simulink model "DM_overflow"  (R2021b)
settings: Solver=FixedStepAuto  StartTime=0.0  StopTime=sim_duration  FixedStep=0.1  RelTol=1e-3
model workspace: external: MAT-File C:\Users\jimmy\Desktop\61508010.mat (data not in the file)
undefined symbols (not defined in the file or in its folder): Base_power, efficiency_3D1, efficiency_3D3, efficiency_speed_3D1, efficiency_speed_3D3, efficiency_torque_3D1, efficiency_torque_3D3, f_d, f_tire_friction, f_tire_speed, g, gear_efficiency, Init_capacity, Max_T_3D1, OCV, OCV_SOC, r_mass, Regen_fraction, Regen_speed, SOC_init, SOC_min, Stop_speed, Torque_curve_speed_3D1, Torque_curve_speed_3D3, Torque_curve_torque_3D1, Torque_curve_torque_3D3, Vehicle_weight, Wheel_radius
libraries: fl_lib x18, nesl_utility x10, sdl_lib x7, simulink x2
settings Model: Creator=jimmy  LastModifiedBy=jimmy
settings DebuggingCC: UnderSpecifiedDimensionMsg=warning
settings SimscapeCC: ExplicitSolverDiagnosticOptions=none

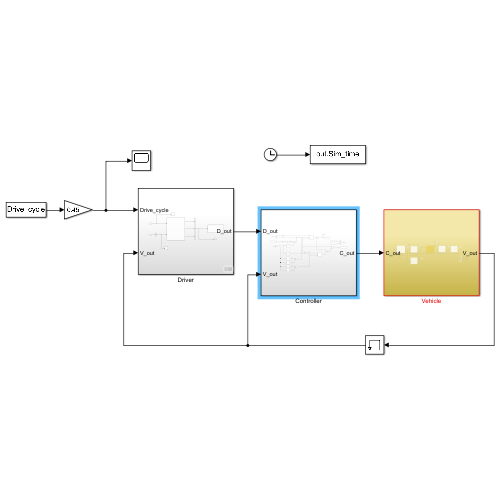
[thumbnail: Simulink's stored preview of the top-level diagram]
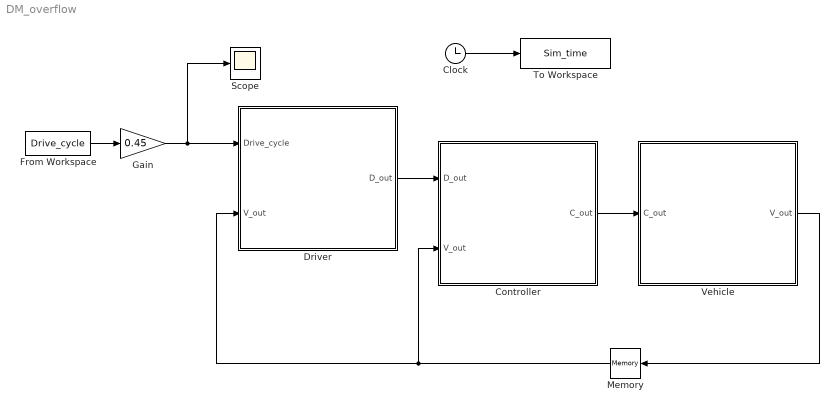
== system DM_overflow ==
  Clock : Clock
  Controller : Subsystem
  Driver : Subsystem
  From Workspace : FromWorkspace  VariableName=Drive_cycle
  Gain : Gain  Gain=0.45
  Memory : Memory  InheritSampleTime=on  LinearizeMemory=on  LinearizeAsDelay=on
  Scope : Scope
  To Workspace : ToWorkspace  VariableName=Sim_time  SaveFormat=Timeseries  SampleTime=-1
  Vehicle : Subsystem
  wires:
  Vehicle/1(V_out) -> Memory/1
  Controller/1(C_out) -> Vehicle/1(C_out)
  Memory/1 -> Controller/2(V_out), Driver/2(V_out)
  Clock/1 -> To Workspace/1
  Driver/1(D_out) -> Controller/1(D_out)
  From Workspace/1 -> Gain/1
  Gain/1 -> Scope/1, Driver/1(Drive_cycle)

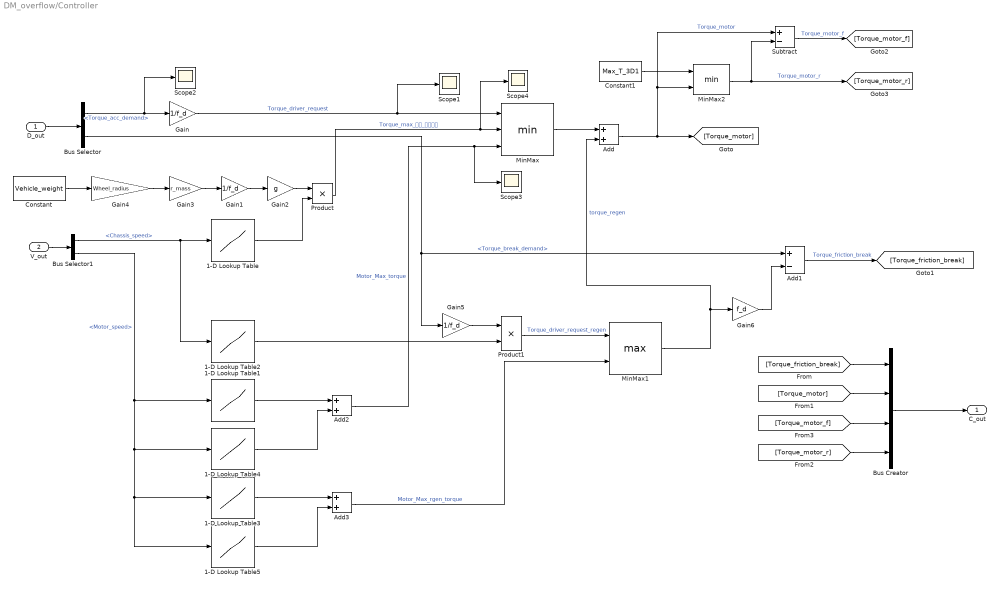
== system DM_overflow/Controller ==
  D_out : Inport
  V_out : Inport  Port=2
  1-D Lookup Table : Lookup_n-D  NumberOfTableDimensions=1  BreakpointsForDimension1=f_tire_speed  Table=f_tire_friction  InternalRulePriority=Speed  RndMeth=Simplest  InputSameDT=on
  1-D Lookup Table1 : Lookup_n-D  NumberOfTableDimensions=1  BreakpointsForDimension1=Torque_curve_speed_3D1  Table=Torque_curve_torque_3D1  InternalRulePriority=Speed  RndMeth=Simplest  InputSameDT=on
  1-D Lookup Table2 : Lookup_n-D  NumberOfTableDimensions=1  BreakpointsForDimension1=Regen_speed  Table=Regen_fraction  InternalRulePriority=Speed  RndMeth=Simplest  InputSameDT=on
  1-D Lookup Table3 : Lookup_n-D  NumberOfTableDimensions=1  BreakpointsForDimension1=Torque_curve_speed_3D1  Table=-Torque_curve_torque_3D1  InternalRulePriority=Speed  RndMeth=Simplest  InputSameDT=on
  1-D Lookup Table4 : Lookup_n-D  NumberOfTableDimensions=1  BreakpointsForDimension1=Torque_curve_speed_3D3  Table=Torque_curve_torque_3D3  InternalRulePriority=Speed  RndMeth=Simplest  InputSameDT=on
  1-D Lookup Table5 : Lookup_n-D  NumberOfTableDimensions=1  BreakpointsForDimension1=Torque_curve_speed_3D3  Table=-Torque_curve_torque_3D3  InternalRulePriority=Speed  RndMeth=Simplest  InputSameDT=on
  Add : Sum
  Add1 : Sum  Inputs=+-
  Add2 : Sum
  Add3 : Sum
  Bus Creator : BusCreator  Inputs=4
  Bus Selector : BusSelector  OutputSignals=Torque_acc_demand,Torque_break_demand
  Bus Selector1 : BusSelector  OutputSignals=Chassis_speed,signal3.Motor_speed
  Constant : Constant  Value=Vehicle_weight
  Constant1 : Constant  Value=Max_T_3D1
  Gain : Gain  Gain=1/f_d
  Gain1 : Gain  Gain=1/f_d
  Gain2 : Gain  Gain=g
  Gain3 : Gain  Gain=r_mass
  Gain4 : Gain  Gain=Wheel_radius
  Gain5 : Gain  Gain=1/f_d
  Gain6 : Gain  Gain=f_d
  MinMax : MinMax  Inputs=3
  MinMax1 : MinMax  Function=max  Inputs=2
  MinMax2 : MinMax  Inputs=2
  Product : Product
  Product1 : Product
  Scope{1..4} (4 alike) : Scope
  Subtract : Sum  Inputs=+-
  C_out : Outport
  wires:
  D_out/1 -> Bus Selector/1
  Bus Selector/1 -> Scope2/1, Gain/1  "<Torque_acc_demand>"
  Bus Selector/2 -> Add1/1, Gain5/1  "<Torque_break_demand>"
  Gain/1 -> Scope1/1, MinMax/1  "Torque_driver_request"
  Constant/1 -> Gain4/1
  Gain4/1 -> Gain3/1
  Gain3/1 -> Gain1/1
  Gain1/1 -> Gain2/1
  1-D Lookup Table/1 -> Product/2
  Bus Selector1/1 -> 1-D Lookup Table2/1, 1-D Lookup Table/1  "<Chassis_speed>"
  Gain2/1 -> Product/1
  V_out/1 -> Bus Selector1/1
  Product/1 -> Scope4/1, MinMax/2  "Torque_max_𝑛𝑜_𝑠𝑙𝑖𝑝"
  MinMax/1 -> Add/1
  Bus Selector1/2 -> 1-D Lookup Table1/1, 1-D Lookup Table4/1, 1-D Lookup Table3/1, 1-D Lookup Table5/1  "<Motor_speed>"
  Gain5/1 -> Product1/1
  1-D Lookup Table2/1 -> Product1/2
  Product1/1 -> MinMax1/1  "Torque_driver_request_regen"
  MinMax1/1 -> Gain6/1, Add/2  "torque_regen"
  Add/1 -> Subtract/1, MinMax2/2, [Torque_motor]  "Torque_motor"
  Gain6/1 -> Add1/2
  Add1/1 -> [Torque_friction_break]  "Torque_friction_break"
  [Torque_motor] -> Bus Creator/2
  [Torque_friction_break] -> Bus Creator/1
  Bus Creator/1 -> C_out/1
  Add3/1 -> MinMax1/2  "Motor_Max_rgen_torque"
  Add2/1 -> Scope3/1, MinMax/3  "Motor_Max_torque"
  1-D Lookup Table1/1 -> Add2/1
  1-D Lookup Table3/1 -> Add3/1
  1-D Lookup Table4/1 -> Add2/2
  1-D Lookup Table5/1 -> Add3/2
  [Torque_motor_f] -> Bus Creator/3
  [Torque_motor_r] -> Bus Creator/4
  Constant1/1 -> MinMax2/1
  MinMax2/1 -> Subtract/2, [Torque_motor_r]  "Torque_motor_r"
  Subtract/1 -> [Torque_motor_f]  "Torque_motor_f"

== system DM_overflow/Driver ==
  Drive_cycle : Inport
  V_out : Inport  Port=2
  Bus Creator : BusCreator  Inputs=3
  Bus Selector : BusSelector  OutputSignals=Chassis_speed
  Plant : Subsystem
  Scope : Scope
  Scope1 : Scope
  To workspace : Subsystem
  D_out : Outport
  wires:
  Drive_cycle/1 -> Scope/1, Plant/1(Drive_cycle)
  V_out/1 -> Bus Selector/1
  Bus Selector/1 -> Scope1/1, Plant/2(Chasis_speed)  "<Chassis_speed>"
  Plant/1(Linear_speed_demand) -> Bus Creator/1
  Plant/2(Torque_acc_demand) -> Bus Creator/2
  Plant/3(Torque_break_demand) -> Bus Creator/3
  Bus Creator/1 -> D_out/1, To workspace/1(In1)

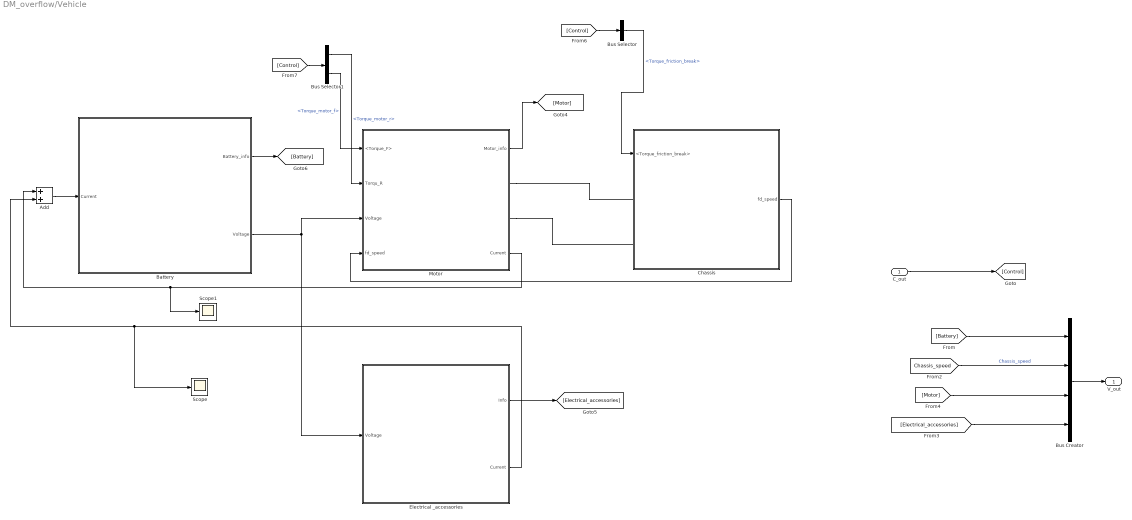
== system DM_overflow/Vehicle ==
  C_out : Inport
  Add : Sum
  Battery : Subsystem
  Bus Creator : BusCreator  Inputs=4
  Bus Selector : BusSelector  OutputSignals=Torque_friction_break
  Bus Selector1 : BusSelector  OutputSignals=Torque_motor_r,Torque_motor_f
  Chassis : Subsystem
  Electrical _accessories : Subsystem
  Motor : Subsystem
      settings: PortSchema="{\"entries\":[{\"content\":{\"sides\":[{\"content\":{\"connectorIds\":[\"In1\",\"In2\",\"In3\",\"In4\"]},\"type\":\"ConnectorPlacement.EquallySpacedRectSide\",\"uuid\":\"41143f5e-7686-4338-be62-9090af3e7fda\"},{\"content\":{\"connectorIds\":[\"Out1\",\"RConn1\",\"RConn2\",\"Out2\"],\"side\":\"RIGHT\"},\"type\":\"ConnectorPlacement.EquallySpacedRectSide\",\"uuid\":\"80376a3c-2384-4fc0-8e0f-19ad3c35f516\"},{\"content\":{\"connectorIds\":[],\"side\":\"TOP\"},\"type\":\"ConnectorPlacement.EquallySpacedRectSide\",\"uuid\":\"cc882acb-b744-4941-b3e2-8b777c6c03a1\"}]},\"type\":\"ConnectorPlacement.EquallySpacedConnector\",\"uuid\":\"b67d3583-afb0-4dd1-8124-18a93feb2c2f\"}],\"packageUris\":[\"http://schema.mathworks.com/mf0/Connector/R2020b\"],\"version\":\"1.0\"}"
  Scope : Scope
  Scope1 : Scope
  V_out : Outport
  wires:
  Bus Creator/1 -> V_out/1
  [Battery] -> Bus Creator/1
  [Chassis_speed] -> Bus Creator/2  "Chassis_speed"
  [Motor] -> Bus Creator/3
  [Electrical_accessories] -> Bus Creator/4
  C_out/1 -> [Control]
  Battery/2(Voltage) -> Motor/3(Voltage), Electrical _accessories/1(Voltage)
  Motor/2(Current) -> Scope1/1, Add/1
  Motor/1(Motor_info) -> [Motor]
  [Control] -> Bus Selector1/1
  Bus Selector1/1 -> Motor/2(Torqu_R)  "<Torque_motor_r>"
  Add/1 -> Battery/1(Current)
  Electrical _accessories/2(Current) -> Scope/1, Add/2
  Electrical _accessories/1(Info) -> [Electrical_accessories]
  Battery/1(Battery_info) -> [Battery]
  Chassis/1(fd_speed) -> Motor/4(fd_speed)
  [Control] -> Bus Selector/1
  Bus Selector/1 -> Chassis/1(<Torque_friction_break>)  "<Torque_friction_break>"
  Bus Selector1/2 -> Motor/1(<Torque_F>)  "<Torque_motor_f>"
  connections:
  Motor/RConn1 -- Chassis/LConn1
  Motor/RConn2 -- Chassis/LConn2

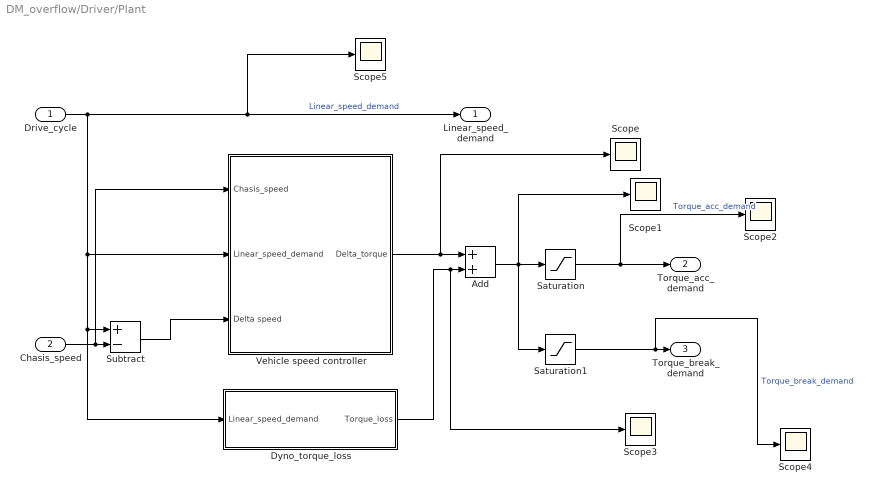
== system DM_overflow/Driver/Plant ==
  Drive_cycle : Inport
  Chasis_speed : Inport  Port=2
  Add : Sum
  Dyno_torque_loss : Subsystem
  Saturation : Saturate  UpperLimit=inf  LowerLimit=0
  Saturation1 : Saturate  UpperLimit=0  LowerLimit=-inf
  Scope{,1..5} (6 alike) : Scope
  Subtract : Sum  Inputs=+-
  Vehicle speed controller : Subsystem
  Linear_speed_demand : Outport
  Torque_acc_demand : Outport  Port=2
  Torque_break_demand : Outport  Port=3
  wires:
  Drive_cycle/1 -> Vehicle speed controller/2(Linear_speed_demand), Dyno_torque_loss/1(Linear_speed_demand), Subtract/1, Scope5/1, Linear_speed_demand/1  "Linear_speed_demand"
  Chasis_speed/1 -> Vehicle speed controller/1(Chasis_speed), Subtract/2
  Subtract/1 -> Vehicle speed controller/3(Delta speed)
  Vehicle speed controller/1(Delta_torque) -> Scope/1, Add/1
  Dyno_torque_loss/1(Torque_loss) -> Scope3/1, Add/2
  Add/1 -> Saturation1/1, Scope1/1, Saturation/1
  Saturation/1 -> Scope2/1, Torque_acc_demand/1  "Torque_acc_demand"
  Saturation1/1 -> Scope4/1, Torque_break_demand/1  "Torque_break_demand"

== system DM_overflow/Driver/To workspace ==
  In1 : Inport
  Bus Selector : BusSelector  OutputSignals=Linear_speed_demand,Torque_acc_demand,Torque_break_demand
  To Workspace : ToWorkspace  VariableName=Linear_speed_demand  SampleTime=0.1
      settings: Decimation=10  Save2DSignal=2-D array (concatenate along first dimension)
  To Workspace2 : ToWorkspace  VariableName=Torque_break_demand  SampleTime=-1
      settings: Decimation=10
  To Workspace3 : ToWorkspace  VariableName=Torque_acc_demand  SampleTime=-1
      settings: Decimation=10
  wires:
  In1/1 -> Bus Selector/1
  Bus Selector/1 -> To Workspace/1  "<Linear_speed_demand>"
  Bus Selector/2 -> To Workspace3/1  "<Torque_acc_demand>"
  Bus Selector/3 -> To Workspace2/1  "<Torque_break_demand>"

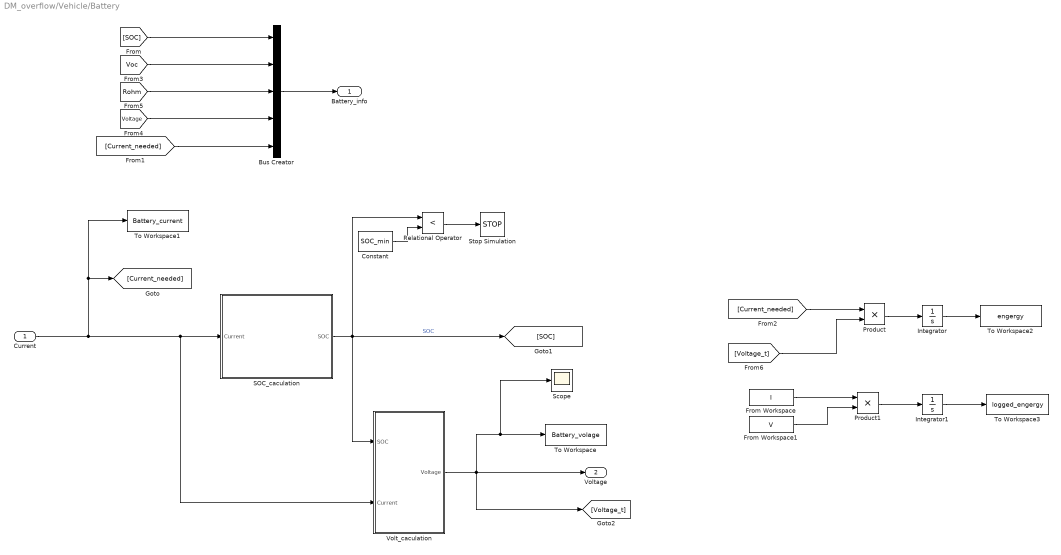
== system DM_overflow/Vehicle/Battery ==
  Current : Inport
  Bus Creator : BusCreator  Inputs=5
  Constant : Constant  Value=SOC_min
  From Workspace : FromWorkspace  VariableName=I
  From Workspace1 : FromWorkspace  VariableName=V
  Integrator : Integrator
  Integrator1 : Integrator
  Product : Product
  Product1 : Product
  Relational Operator : RelationalOperator  Operator=<  OutDataTypeStr=boolean  RndMeth=Simplest
  SOC_caculation : Subsystem
  Scope : Scope
  Stop Simulation : Stop
  To Workspace : ToWorkspace  VariableName=Battery_volage  SampleTime=0.1
  To Workspace1 : ToWorkspace  VariableName=Battery_current  SampleTime=0.1
  To Workspace2 : ToWorkspace  VariableName=engergy  SampleTime=-1
  To Workspace3 : ToWorkspace  VariableName=logged_engergy  SampleTime=-1
  Volt_caculation : Subsystem
  Battery_info : Outport
  Voltage : Outport  Port=2
  wires:
  Current/1 -> To Workspace1/1, [Current_needed], Volt_caculation/2(Current), SOC_caculation/1(Current)
  SOC_caculation/1(SOC) -> Volt_caculation/1(SOC), Relational Operator/1, [SOC]  "SOC"
  Constant/1 -> Relational Operator/2
  Relational Operator/1 -> Stop Simulation/1
  Volt_caculation/1(Voltage) -> [Voltage_t], Scope/1, To Workspace/1, Voltage/1
  Bus Creator/1 -> Battery_info/1
  [Current_needed] -> Bus Creator/5
  [SOC] -> Bus Creator/1
  [Voc] -> Bus Creator/2
  [Rohm] -> Bus Creator/3
  [Voltage] -> Bus Creator/4
  [Voltage_t] -> Product/2
  [Current_needed] -> Product/1
  Product/1 -> Integrator/1
  Integrator/1 -> To Workspace2/1
  From Workspace/1 -> Product1/1
  From Workspace1/1 -> Product1/2
  Product1/1 -> Integrator1/1
  Integrator1/1 -> To Workspace3/1

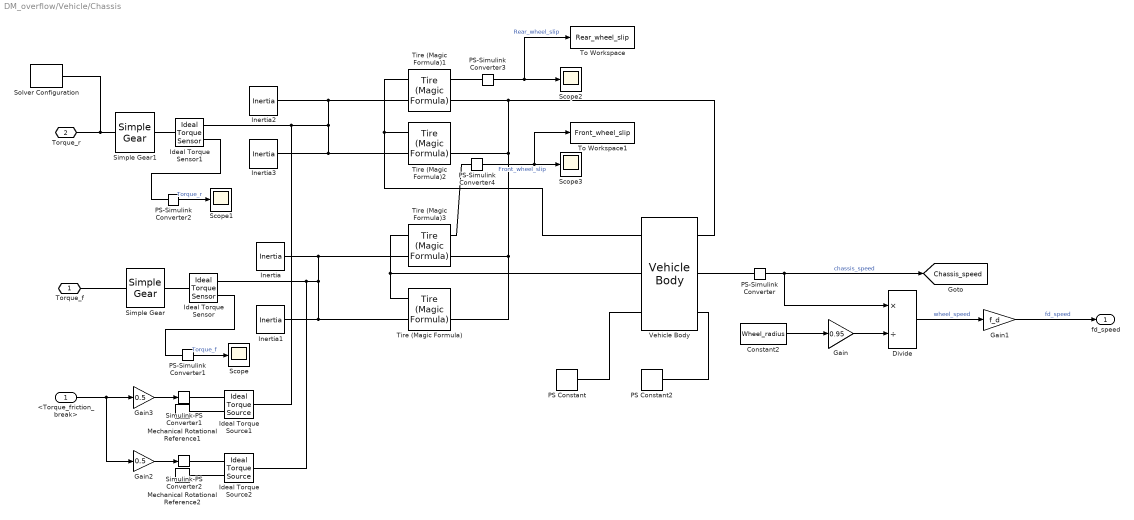
== system DM_overflow/Vehicle/Chassis ==
  <Torque_friction_break> : Inport
  Constant2 : Constant  Value=Wheel_radius
  Divide : Product  Inputs=*/
  Gain : Gain  Gain=0.95
  Gain1 : Gain  Gain=f_d
  Gain2 : Gain  Gain=0.5
  Gain3 : Gain  Gain=0.5
  Ideal Torque Sensor : fl_lib/Mechanical/Mechanical Sensors/Ideal Torque Sensor
  Ideal Torque Sensor1 : fl_lib/Mechanical/Mechanical Sensors/Ideal Torque Sensor
  Ideal Torque Source1 : fl_lib/Mechanical/Mechanical Sources/Ideal Torque Source
  Ideal Torque Source2 : fl_lib/Mechanical/Mechanical Sources/Ideal Torque Source
  Inertia{,1..3} (4 alike) : fl_lib/Mechanical/Rotational Elements/Inertia  inertia=1 kg*m^2  num_ports=foundation.enum.numPorts2.one  w_specify=off  w_priority=High  w=0 rad/s  w_nominal_specify=off  w_nominal_unit=rad/s  w_nominal_value=1  t_specify=off  t_priority=None  t=0 N*m  t_nominal_specify=off  t_nominal_unit=N*m  t_nominal_value=1
  Mechanical Rotational Reference1 : fl_lib/Mechanical/Rotational Elements/Mechanical Rotational Reference
  Mechanical Rotational Reference2 : fl_lib/Mechanical/Rotational Elements/Mechanical Rotational Reference
  PS Constant : fl_lib/Physical Signals/Sources/PS Constant  constant=0
  PS Constant2 : fl_lib/Physical Signals/Sources/PS Constant  constant=5 m/s
  PS-Simulink Converter{,1..4} (5 alike) : nesl_utility/PS-Simulink Converter  PhysicalDomain=network_engine_domain  SubClassName=ps_output  LeftPortType=input  RightPortType=output  PseudoPeriodic=off  Frequencies=[]  Unit=inherit  AffineConversion=off
      settings: SourceProductBaseCode=PW,SS
  Scope{,1..3} (4 alike) : Scope
  Simple Gear : sdl_lib/Gears/Simple Gear  ratio=f_d  rotation_direction=sdl.enum.shaftOutputDirection.same  friction_model=sdl.enum.gear_efficiencies_load.off  T_noload=0.1 N*m  T_nom=5 N*m  efficiency_nom=0.8  efficiency=0.8  temperature_TLU=[280, 300, 320] K  load_TLU=[1, 5, 10] N*m  efficiency_TLU=[.95, .9, .85]  efficiency_TLU2=[.85, .8, .75; .95, .9, .85; .85, .8, .7]  w_thr=0.01 rad/s  pwr_thr=0.001 W  backlash_model=sdl.enum.backlashModel.Off  backlash_distance=1e-3 mm  x0=0 mm  r_base=0.1 m  hardstop_model=simscape.enum.hardstop.smooth  transition=1e-4 mm  backlash_stiffness=1e7 N/m  backlash_damping=1e6 N/(m/s)  e=0  v_tol=0.001 m/s  mu_visc=[0, 0] N*m/(rad/s)  enable_faults=simscape.enum.onoff.off  efficiency_fault=0.05  external_fault=simscape.enum.onoff.off  temporal_fault=simscape.enum.onoff.off  fault_time=5 s  fault_angles=pi / 12 rad  report_fault=simscape.enum.assert.action.none  thermal_mass=50 J/K  temperature_specify=off  temperature_priority=High  temperature=300 K  temperature_nominal_specify=off  temperature_nominal_unit=K  temperature_nominal_value=1  x_backlash_specify=off  x_backlash_priority=None  x_backlash=0 mm  x_backlash_nominal_specify=off  x_backlash_nominal_unit=mm  x_backlash_nominal_value=1  f_hardstop_specify=off  f_hardstop_priority=None  f_hardstop=0 N  f_hardstop_nominal_specify=off  f_hardstop_nominal_unit=N  f_hardstop_nominal_value=1  v_backlash_specify=off  v_backlash_priority=None  v_backlash=0 m/s  v_backlash_nominal_specify=off  v_backlash_nominal_unit=m/s  v_backlash_nominal_value=1
  Simple Gear1 : sdl_lib/Gears/Simple Gear  ratio=f_d  rotation_direction=sdl.enum.shaftOutputDirection.same  friction_model=sdl.enum.gear_efficiencies_load.off  T_noload=0.1 N*m  T_nom=5 N*m  efficiency_nom=0.8  efficiency=0.8  temperature_TLU=[280, 300, 320] K  load_TLU=[1, 5, 10] N*m  efficiency_TLU=[.95, .9, .85]  efficiency_TLU2=[.85, .8, .75; .95, .9, .85; .85, .8, .7]  w_thr=0.01 rad/s  pwr_thr=0.001 W  backlash_model=sdl.enum.backlashModel.Off  backlash_distance=1e-3 mm  x0=0 mm  r_base=0.1 m  hardstop_model=simscape.enum.hardstop.smooth  transition=1e-4 mm  backlash_stiffness=1e7 N/m  backlash_damping=1e6 N/(m/s)  e=0  v_tol=0.001 m/s  mu_visc=[0, 0] N*m/(rad/s)  enable_faults=simscape.enum.onoff.off  efficiency_fault=0.05  external_fault=simscape.enum.onoff.off  temporal_fault=simscape.enum.onoff.off  fault_time=5 s  fault_angles=pi / 12 rad  report_fault=simscape.enum.assert.action.none  thermal_mass=50 J/K  temperature_specify=off  temperature_priority=High  temperature=300 K  temperature_nominal_specify=off  temperature_nominal_unit=K  temperature_nominal_value=1  x_backlash_specify=off  x_backlash_priority=None  x_backlash=0 mm  x_backlash_nominal_specify=off  x_backlash_nominal_unit=mm  x_backlash_nominal_value=1  f_hardstop_specify=off  f_hardstop_priority=None  f_hardstop=0 N  f_hardstop_nominal_specify=off  f_hardstop_nominal_unit=N  f_hardstop_nominal_value=1  v_backlash_specify=off  v_backlash_priority=None  v_backlash=0 m/s  v_backlash_nominal_specify=off  v_backlash_nominal_unit=m/s  v_backlash_nominal_value=1
  Simulink-PS Converter1 : nesl_utility/Simulink-PS Converter  PhysicalDomain=network_engine_domain  SubClassName=ps_input  LeftPortType=input  RightPortType=output  PseudoPeriodic=off  Frequencies=[]  NoiseDistribution=none  NoiseParameters=[]  Unit=N*m  AffineConversion=off  FilteringAndDerivatives=provide  SimscapeFilterOrder=2  InputFilterTimeConstant=0.001  UdotUserProvided=0
      settings: SourceProductBaseCode=PW,SS
  Simulink-PS Converter2 : nesl_utility/Simulink-PS Converter  PhysicalDomain=network_engine_domain  SubClassName=ps_input  LeftPortType=input  RightPortType=output  PseudoPeriodic=off  Frequencies=[]  NoiseDistribution=none  NoiseParameters=[]  Unit=N*m  AffineConversion=off  FilteringAndDerivatives=provide  SimscapeFilterOrder=2  InputFilterTimeConstant=0.001  UdotUserProvided=0
      settings: SourceProductBaseCode=PW,SS
  Solver Configuration : nesl_utility/Solver Configuration  PhysicalDomain=network_engine_domain  SubClassName=solver  LeftPortType=input  RightPortType=generic  Tones=[]  Harmonics=[]  SimulateNoise=off  Profile=off  UseLocalSampling=off  EnableSwitchedLinearOptims=on  FrequencyDomain=off  UseCCode=off  RelTol=0.001  AbsTol=1e-06  MinStep=1e-09  ToWorkspace=off  RevertToSquareIcSolve=off  NumHomotopyIterations=100  PhasorMode=off  PhasorModeNumHarmonics=1  DoDC=off  ResidualTolerance=1e-06  UseLocalSolver=off  LocalSolverChoice=NE_BACKWARD_EULER_ADVANCER  LocalSolverSampleTime=0.001  DoFixedCost=off  MaxNonlinIter=3  MaxModeIter=2  ComputeImpulses=off  ImpulseIterations=2  LinearAlgebra=auto  EquationFormulation=NE_TIME_EF  DelaysMemoryBudget=1024  AutomaticFiltering=on  FilteringTimeConstant=0.01  PartitionStorageMethod=AS_NEEDED  PartitionMemoryBudget=1024  PartitionMethod=ROBUST
      settings: SourceProductBaseCode=PW,SS
  Tire (Magic Formula){,1..3} (4 alike) : sdl_lib/Tires & Vehicles/Tire (Magic Formula)  parameterization=sdl.enum.magic_tire_model.constant  F_z1=3000 N  F_x1=3500 N  kappa1=10  B_m=10  C_m=1.9  D_m=1  E_m=0.97  fz0=4000 N  p_Cx=1.685  p_Dx=[1.21, -.037]  p_Ex=[.344, .095, -.02, 0]  p_Kx=[21.51, -.163, .245]  p_Hx=[-.002, .002]  p_Vx=[0, 0]  r_e=Wheel_radius m  model_compliance=sdl.enum.compliance.off  stiffness=1e6 N/m  damping=1000 N/(m/s)  model_inertia=sdl.enum.model_inertia.on  inertia=1 kg*m^2  initial_velocity=0 rad/s  model_resistance=simscape.enum.onoff.on  resistance_model=sdl.enum.rollingResistanceParameterization.constant  coeff=0.015  p_tire=250e3 Pa  alpha=-0.003  beta=0.97  coeff_a=84e-4  coeff_b=6.2e-4 s/m  coeff_c=1.6e-4 s^2/m^2  v_thr=0.001 m/s  v_tr_thr=0.1 m/s
  To Workspace : ToWorkspace  VariableName=Rear_wheel_slip  SampleTime=-1
  To Workspace1 : ToWorkspace  VariableName=Front_wheel_slip  SampleTime=-1
  Vehicle Body : sdl_lib/Tires & Vehicles/Vehicle Body  mass=Vehicle_weight kg  n_w=2  x_f=CG_f mm  x_r=CG_r mm  y_c=CG_h mm  mass_var=simscape.enum.onoff.off  g=9.81 m/s^2  liftoff_warning=simscape.enum.onoff.off  area=2.48 m^2  Cd=0.4  rho=1.23 kg/m^3  model_pitch=simscape.enum.onoff.off  inertia=4000 kg*m^2  suspension_model=sdl.enum.linearTLU.linear  k_f=1e4 N/m  b_f=1e4 N/(m/s)  k_r=1e4 N/m  b_r=1e4 N/(m/s)  k_f_TLU=[-2000, -1000, 0, 1000, 2000] N  x_f_TLU=[-.4, -.2, 0, .2, .4] m  b_f_TLU=[-200, -100, 0, 100, 200] N  v_f_TLU=[-4, -2, 0, 2, 4] m/s  k_r_TLU=[-2000, -1000, 0, 1000, 2000] N  x_r_TLU=[-.4, -.2, 0, .2, .4] m  b_r_TLU=[-200, -100, 0, 100, 200] N  v_r_TLU=[-4, -2, 0, 2, 4] m/s  interp_method=simscape.enum.interpolation.linear  extrap_method=simscape.enum.extrapolation.linear  model_hardstop=simscape.enum.onoff.off  upper_bound_f=.25 m  lower_bound_f=-.25 m  stop_k_f=1e6 N/m  stop_b_f=150 N/(m/s)  upper_bound_r=.25 m  lower_bound_r=-.25 m  stop_k_r=1e6 N/m  stop_b_r=150 N/(m/s)  initial_pitch=0 rad  initial_pitch_rate=0 rad/s  v_specify=off  v_priority=High  v=0 m/s  v_nominal_specify=off  v_nominal_unit=m/s  v_nominal_value=1
  Torque_f : PMIOPort  Side=Left
  Torque_r : PMIOPort  Port=2  Side=Left
  fd_speed : Outport
  tag scope: Chassis_speed=global
  wires:
  PS-Simulink Converter/1 -> Divide/1, [Chassis_speed]  "chassis_speed"
  Constant2/1 -> Gain/1
  Gain/1 -> Divide/2
  Divide/1 -> Gain1/1  "wheel_speed"
  Gain1/1 -> fd_speed/1  "fd_speed"
  PS-Simulink Converter1/1 -> Scope/1  "Torque_f"
  PS-Simulink Converter2/1 -> Scope1/1  "Torque_r"
  PS-Simulink Converter3/1 -> To Workspace/1, Scope2/1  "Rear_wheel_slip"
  PS-Simulink Converter4/1 -> To Workspace1/1, Scope3/1  "Front_wheel_slip"
  Gain3/1 -> Simulink-PS Converter1/1
  <Torque_friction_break>/1 -> Gain2/1, Gain3/1
  Gain2/1 -> Simulink-PS Converter2/1
  connections:
  Vehicle Body/RConn1 -- Tire (Magic Formula)1/LConn1 -- Tire (Magic Formula)2/LConn1
  Vehicle Body/RConn2 -- Tire (Magic Formula)3/LConn1 -- Tire (Magic Formula)/LConn1
  Tire (Magic Formula)/LConn2 -- Inertia1/LConn1 -- Ideal Torque Source2/LConn1 -- Ideal Torque Sensor/RConn1 -- Tire (Magic Formula)3/LConn2 -- Inertia/LConn1
  Tire (Magic Formula)3/RConn2 -- Tire (Magic Formula)/RConn2 -- Tire (Magic Formula)2/RConn2 -- Tire (Magic Formula)1/RConn2 -- Vehicle Body/LConn1
  Vehicle Body/LConn2 -- PS-Simulink Converter/LConn1
  Inertia3/LConn1 -- Tire (Magic Formula)2/LConn2 -- Ideal Torque Source1/LConn1 -- Ideal Torque Sensor1/RConn1 -- Tire (Magic Formula)1/LConn2 -- Inertia2/LConn1
  Torque_r/RConn1 -- Solver Configuration/RConn1 -- Simple Gear1/LConn1
  Torque_f/RConn1 -- Simple Gear/LConn1
  Simple Gear/RConn1 -- Ideal Torque Sensor/LConn1
  Ideal Torque Sensor/RConn2 -- PS-Simulink Converter1/LConn1
  Ideal Torque Sensor1/RConn2 -- PS-Simulink Converter2/LConn1
  Simple Gear1/RConn1 -- Ideal Torque Sensor1/LConn1
  PS-Simulink Converter3/LConn1 -- Tire (Magic Formula)1/RConn1
  PS-Simulink Converter4/LConn1 -- Tire (Magic Formula)3/RConn1
  PS Constant/RConn1 -- Vehicle Body/RConn3
  Mechanical Rotational Reference1/LConn1 -- Ideal Torque Source1/RConn2
  Simulink-PS Converter1/RConn1 -- Ideal Torque Source1/RConn1
  Simulink-PS Converter2/RConn1 -- Ideal Torque Source2/RConn1
  Mechanical Rotational Reference2/LConn1 -- Ideal Torque Source2/RConn2
  PS Constant2/RConn1 -- Vehicle Body/LConn3

== system DM_overflow/Vehicle/Electrical _accessories ==
  Voltage : Inport
  Constant : Constant  Value=Base_power
  Divider : Subsystem
  Info : Outport
  Current : Outport  Port=2
  wires:
  Divider/1(Out1) -> Current/1
  Constant/1 -> Divider/1(Current)
  Voltage/1 -> Divider/2(Voltage)

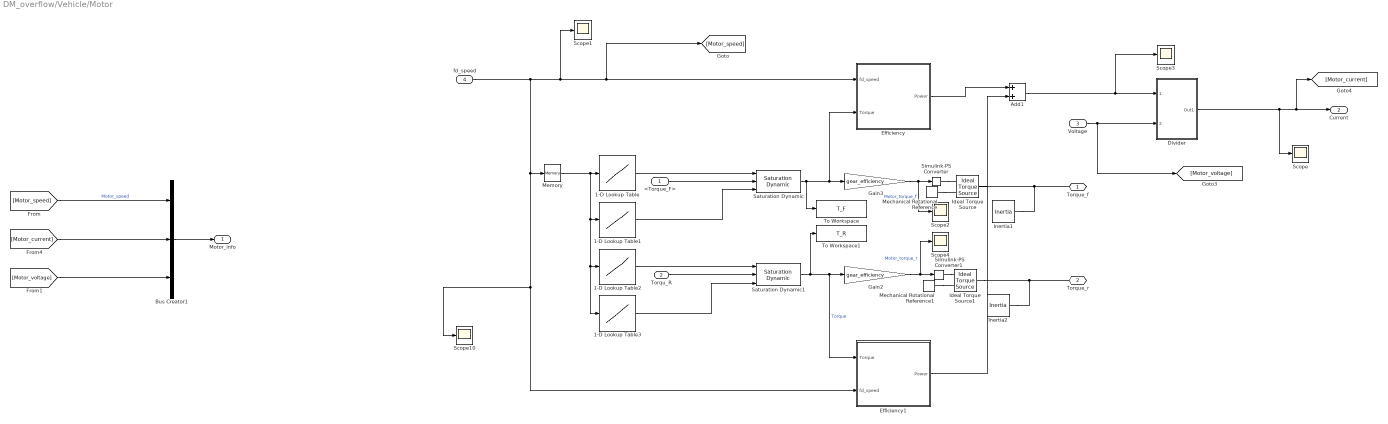
== system DM_overflow/Vehicle/Motor ==
  <Torque_F> : Inport
  Torqu_R : Inport  Port=2
  Voltage : Inport  Port=3
  fd_speed : Inport  Port=4
  1-D Lookup Table : Lookup_n-D  NumberOfTableDimensions=1  BreakpointsForDimension1=Torque_curve_speed_3D3  Table=Torque_curve_torque_3D3  InternalRulePriority=Speed  RndMeth=Simplest  InputSameDT=on
  1-D Lookup Table1 : Lookup_n-D  NumberOfTableDimensions=1  BreakpointsForDimension1=Torque_curve_speed_3D3  Table=-Torque_curve_torque_3D3  InternalRulePriority=Speed  RndMeth=Simplest  InputSameDT=on
  1-D Lookup Table2 : Lookup_n-D  NumberOfTableDimensions=1  BreakpointsForDimension1=Torque_curve_speed_3D1  Table=Torque_curve_torque_3D1  InternalRulePriority=Speed  RndMeth=Simplest  InputSameDT=on
  1-D Lookup Table3 : Lookup_n-D  NumberOfTableDimensions=1  BreakpointsForDimension1=Torque_curve_speed_3D1  Table=-Torque_curve_torque_3D1  InternalRulePriority=Speed  RndMeth=Simplest  InputSameDT=on
  Add1 : Sum
  Bus Creator1 : BusCreator  Inputs=3
  Divider : Subsystem
  Efficiency : Subsystem
  Efficiency1 : Subsystem
  Gain2 : Gain  Gain=gear_efficiency
  Gain3 : Gain  Gain=gear_efficiency
  Ideal Torque Source : fl_lib/Mechanical/Mechanical Sources/Ideal Torque Source
  Ideal Torque Source1 : fl_lib/Mechanical/Mechanical Sources/Ideal Torque Source
  Inertia1 : fl_lib/Mechanical/Rotational Elements/Inertia  inertia=1 kg*m^2  num_ports=foundation.enum.numPorts2.one  w_specify=off  w_priority=High  w=0 rad/s  w_nominal_specify=off  w_nominal_unit=rad/s  w_nominal_value=1  t_specify=off  t_priority=None  t=0 N*m  t_nominal_specify=off  t_nominal_unit=N*m  t_nominal_value=1
  Inertia2 : fl_lib/Mechanical/Rotational Elements/Inertia  inertia=1 kg*m^2  num_ports=foundation.enum.numPorts2.one  w_specify=off  w_priority=High  w=0 rad/s  w_nominal_specify=off  w_nominal_unit=rad/s  w_nominal_value=1  t_specify=off  t_priority=None  t=0 N*m  t_nominal_specify=off  t_nominal_unit=N*m  t_nominal_value=1
  Mechanical Rotational Reference : fl_lib/Mechanical/Rotational Elements/Mechanical Rotational Reference
  Mechanical Rotational Reference1 : fl_lib/Mechanical/Rotational Elements/Mechanical Rotational Reference
  Memory : Memory  InheritSampleTime=on  LinearizeMemory=on  LinearizeAsDelay=on
  Saturation Dynamic : simulink/Discontinuities/Saturation Dynamic  OutMin=[]  OutMax=[]  OutDataTypeStr=Inherit: Same as second input  OutDataType=fixdt(1, 16)  OutScaling=2^-10  DoSatur=off
  Saturation Dynamic1 : simulink/Discontinuities/Saturation Dynamic  OutMin=[]  OutMax=[]  OutDataTypeStr=Inherit: Same as second input  OutDataType=fixdt(1, 16)  OutScaling=2^-10  DoSatur=off
  Scope{,1..4,10} (6 alike) : Scope
  Simulink-PS Converter : nesl_utility/Simulink-PS Converter  PhysicalDomain=network_engine_domain  SubClassName=ps_input  LeftPortType=input  RightPortType=output  PseudoPeriodic=off  Frequencies=[]  NoiseDistribution=none  NoiseParameters=[]  Unit=N*m  AffineConversion=off  FilteringAndDerivatives=provide  SimscapeFilterOrder=2  InputFilterTimeConstant=0.001  UdotUserProvided=0
      settings: SourceProductBaseCode=PW,SS
  Simulink-PS Converter1 : nesl_utility/Simulink-PS Converter  PhysicalDomain=network_engine_domain  SubClassName=ps_input  LeftPortType=input  RightPortType=output  PseudoPeriodic=off  Frequencies=[]  NoiseDistribution=none  NoiseParameters=[]  Unit=N*m  AffineConversion=off  FilteringAndDerivatives=provide  SimscapeFilterOrder=2  InputFilterTimeConstant=0.01  UdotUserProvided=0
      settings: SourceProductBaseCode=PW,SS
  To Workspace : ToWorkspace  VariableName=T_F  SampleTime=-1
  To Workspace1 : ToWorkspace  VariableName=T_R  SampleTime=-1
  Torque_f : PMIOPort  Side=Right
  Torque_r : PMIOPort  Port=2  Side=Right
  Motor_info : Outport
  Current : Outport  Port=2
  wires:
  Memory/1 -> 1-D Lookup Table1/1, 1-D Lookup Table2/1, 1-D Lookup Table3/1, 1-D Lookup Table/1
  1-D Lookup Table1/1 -> Saturation Dynamic/3
  Voltage/1 -> [Motor_voltage], Divider/2(2)
  Divider/1(Out1) -> Current/1, [Motor_current], Scope/1
  [Motor_speed] -> Bus Creator1/1  "Motor_speed"
  [Motor_current] -> Bus Creator1/2
  fd_speed/1 -> Scope10/1, Efficiency1/2(fd_speed), Memory/1, Scope1/1, [Motor_speed], Efficiency/1(fd_speed)
  1-D Lookup Table/1 -> Saturation Dynamic/1
  [Motor_voltage] -> Bus Creator1/3
  Bus Creator1/1 -> Motor_info/1
  1-D Lookup Table2/1 -> Saturation Dynamic1/1
  1-D Lookup Table3/1 -> Saturation Dynamic1/3
  Efficiency1/1(Power) -> Add1/2
  Add1/1 -> Divider/1(1), Scope3/1
  Efficiency/1(Power) -> Add1/1
  Gain2/1 -> Scope4/1, Simulink-PS Converter1/1  "Motor_torque_r"
  Gain3/1 -> Scope2/1, Simulink-PS Converter/1  "Motor_torque_f"
  <Torque_F>/1 -> Saturation Dynamic/2
  Torqu_R/1 -> Saturation Dynamic1/2
  Saturation Dynamic/1 -> To Workspace/1, Efficiency/2(Torque), Gain3/1
  Saturation Dynamic1/1 -> To Workspace1/1, Efficiency1/1(Torque), Gain2/1  "Torque"
  connections:
  Simulink-PS Converter/RConn1 -- Ideal Torque Source/RConn1
  Mechanical Rotational Reference/LConn1 -- Ideal Torque Source/RConn2
  Ideal Torque Source/LConn1 -- Inertia1/LConn1 -- Torque_f/RConn1
  Ideal Torque Source1/LConn1 -- Torque_r/RConn1 -- Inertia2/LConn1
  Simulink-PS Converter1/RConn1 -- Ideal Torque Source1/RConn1
  Mechanical Rotational Reference1/LConn1 -- Ideal Torque Source1/RConn2

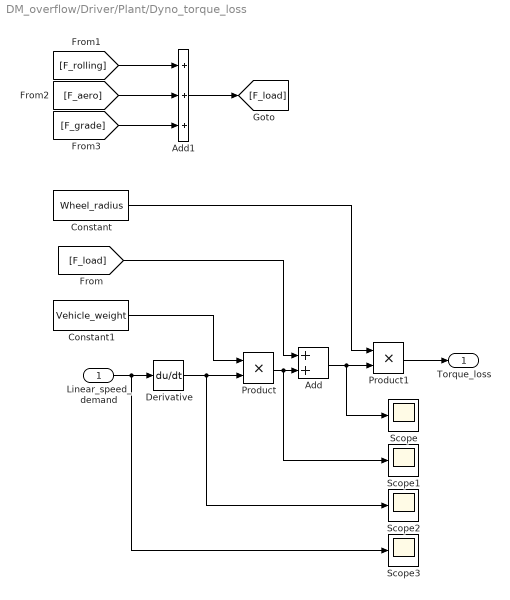
== system DM_overflow/Driver/Plant/Dyno_torque_loss ==
  Linear_speed_demand : Inport
  Add : Sum
  Add1 : Sum  Inputs=+++
  Constant : Constant  Value=Wheel_radius
  Constant1 : Constant  Value=Vehicle_weight
  Derivative : Derivative
  Product : Product
  Product1 : Product
  Scope{,1..3} (4 alike) : Scope
  Torque_loss : Outport
  wires:
  Linear_speed_demand/1 -> Scope3/1, Derivative/1
  Derivative/1 -> Scope2/1, Product/2
  Constant1/1 -> Product/1
  Product/1 -> Scope1/1, Add/2
  [F_load] -> Add/1
  Add/1 -> Scope/1, Product1/2
  Constant/1 -> Product1/1
  Product1/1 -> Torque_loss/1
  [F_rolling] -> Add1/1
  [F_aero] -> Add1/2
  [F_grade] -> Add1/3
  Add1/1 -> [F_load]

== system DM_overflow/Driver/Plant/Vehicle speed controller ==
  Chasis_speed : Inport
  Linear_speed_demand : Inport  Port=2
  Delta speed : Inport  Port=3
  Add : Sum
  Constant : Constant  Value=Stop_speed
  I : Gain  Gain=0.5
  Integrator : Integrator  ExternalReset=either
  P : Gain  Gain=1000
  Relational Operator : RelationalOperator  Operator=<  OutDataTypeStr=boolean  RndMeth=Simplest
  Delta_torque : Outport
  wires:
  Delta speed/1 -> P/1, Integrator/1
  Chasis_speed/1 -> Relational Operator/1
  Constant/1 -> Relational Operator/2
  Relational Operator/1 -> Integrator/2
  Integrator/1 -> I/1
  P/1 -> Add/1
  I/1 -> Add/2
  Add/1 -> Delta_torque/1  "Delta_torque"

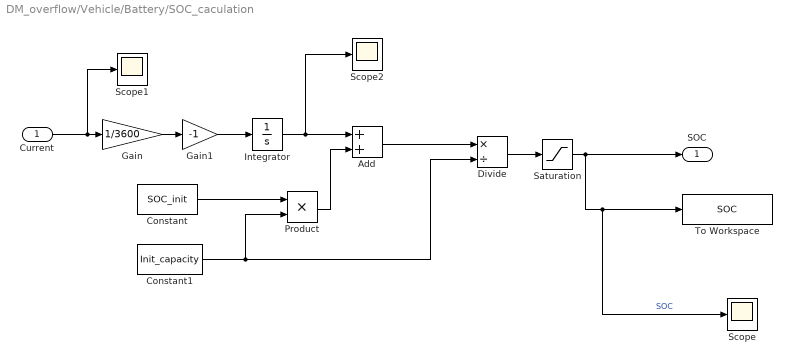
== system DM_overflow/Vehicle/Battery/SOC_caculation ==
  Current : Inport
  Add : Sum
  Constant : Constant  Value=SOC_init
  Constant1 : Constant  Value=Init_capacity
  Divide : Product  Inputs=*/
  Gain : Gain  Gain=1/3600
  Gain1 : Gain  Gain=-1
  Integrator : Integrator
  Product : Product
  Saturation : Saturate  UpperLimit=1  LowerLimit=0
  Scope : Scope
  Scope1 : Scope
  Scope2 : Scope
  To Workspace : ToWorkspace  VariableName=SOC  SampleTime=0.1
  SOC : Outport
  wires:
  Gain/1 -> Gain1/1
  Current/1 -> Scope1/1, Gain/1
  Gain1/1 -> Integrator/1
  Constant/1 -> Product/1
  Constant1/1 -> Divide/2, Product/2
  Divide/1 -> Saturation/1
  Add/1 -> Divide/1
  Integrator/1 -> Scope2/1, Add/1
  Product/1 -> Add/2
  Saturation/1 -> Scope/1, To Workspace/1, SOC/1  "SOC"

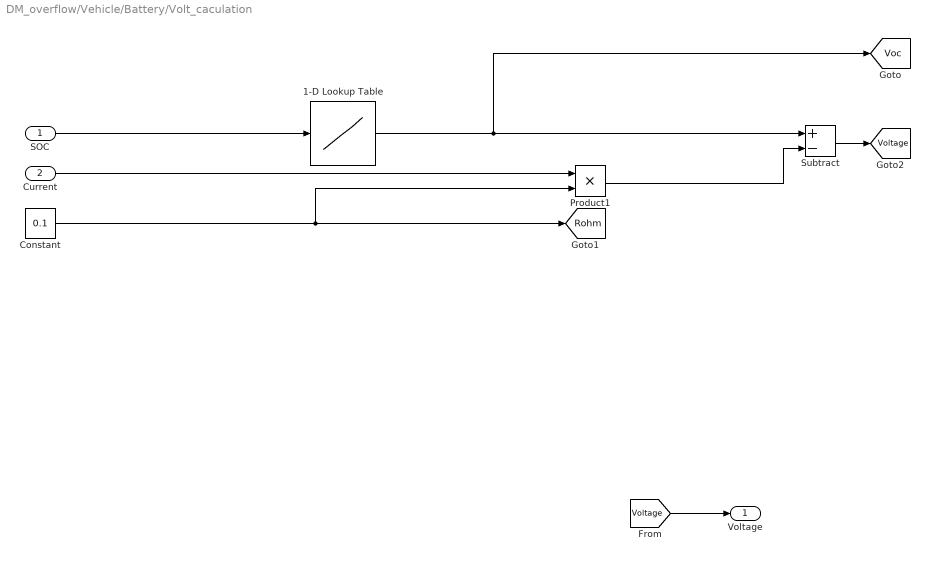
== system DM_overflow/Vehicle/Battery/Volt_caculation ==
  SOC : Inport
  Current : Inport  Port=2
  1-D Lookup Table : Lookup_n-D  NumberOfTableDimensions=1  BreakpointsForDimension1=OCV_SOC  Table=OCV  InternalRulePriority=Speed  RndMeth=Simplest  InputSameDT=on
  Constant : Constant  Value=0.1
  Product1 : Product
  Subtract : Sum  Inputs=+-
  Voltage : Outport
  tag scope: Rohm=global, Voc=global, Voltage=global
  wires:
  SOC/1 -> 1-D Lookup Table/1
  1-D Lookup Table/1 -> Subtract/1, [Voc]
  Constant/1 -> [Rohm], Product1/2
  Current/1 -> Product1/1
  Product1/1 -> Subtract/2
  Subtract/1 -> [Voltage]
  [Voltage] -> Voltage/1

== system DM_overflow/Vehicle/Electrical _accessories/Divider ==
  Current : Inport
  Voltage : Inport  Port=2
  Bus Creator : BusCreator  Inputs=2
  Interpreted MATLAB Function : MATLABFcn  MATLABFcn=myFunction
  Out1 : Outport
  wires:
  Current/1 -> Bus Creator/1
  Voltage/1 -> Bus Creator/2
  Bus Creator/1 -> Interpreted MATLAB Function/1
  Interpreted MATLAB Function/1 -> Out1/1

== system DM_overflow/Vehicle/Motor/Divider ==
  1 : Inport
  2 : Inport  Port=2
  Bus Creator : BusCreator  Inputs=2
  Interpreted MATLAB Function : MATLABFcn  MATLABFcn=myFunction
  Out1 : Outport
  wires:
  1/1 -> Bus Creator/1
  2/1 -> Bus Creator/2
  Bus Creator/1 -> Interpreted MATLAB Function/1
  Interpreted MATLAB Function/1 -> Out1/1

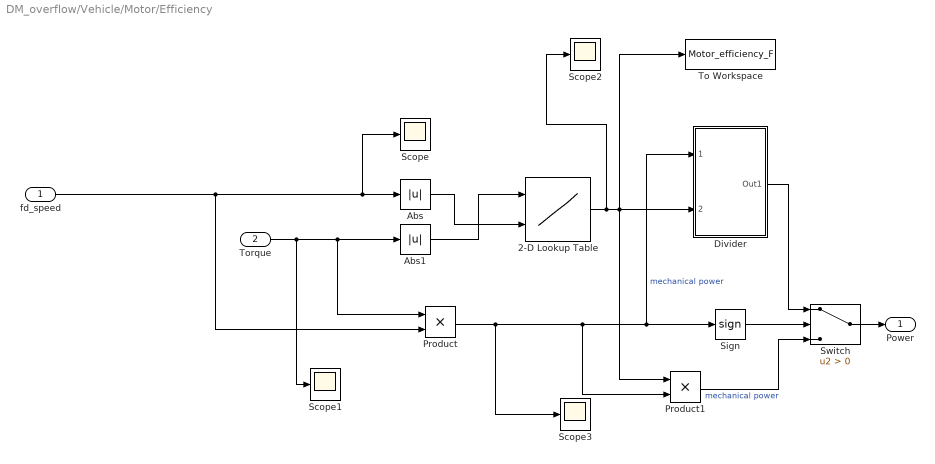
== system DM_overflow/Vehicle/Motor/Efficiency ==
  fd_speed : Inport
  Torque : Inport  Port=2
  2-D Lookup Table : Lookup_n-D  BreakpointsForDimension1=efficiency_torque_3D3  BreakpointsForDimension2=efficiency_speed_3D3  Table=efficiency_3D3  InternalRulePriority=Speed  RndMeth=Simplest  InputSameDT=on
      settings: InputPortMap=u0,u1
  Abs : Abs
  Abs1 : Abs
  Divider : Subsystem
  Product : Product
  Product1 : Product
  Scope{,1..3} (4 alike) : Scope
  Sign : Signum
  Switch : Switch  Criteria=u2 > Threshold
  To Workspace : ToWorkspace  VariableName=Motor_efficiency_F  SaveFormat=Timeseries  SampleTime=-1
  Power : Outport
  wires:
  Torque/1 -> Scope1/1, Product/1, Abs1/1
  Product/1 -> Scope3/1, Product1/2, Divider/1(1), Sign/1  "mechanical power"
  Sign/1 -> Switch/2
  Switch/1 -> Power/1
  2-D Lookup Table/1 -> Scope2/1, Product1/1, To Workspace/1, Divider/2(2)
  Product1/1 -> Switch/3  "mechanical power"
  Divider/1(Out1) -> Switch/1
  Abs1/1 -> 2-D Lookup Table/1
  Abs/1 -> 2-D Lookup Table/2
  fd_speed/1 -> Scope/1, Abs/1, Product/2

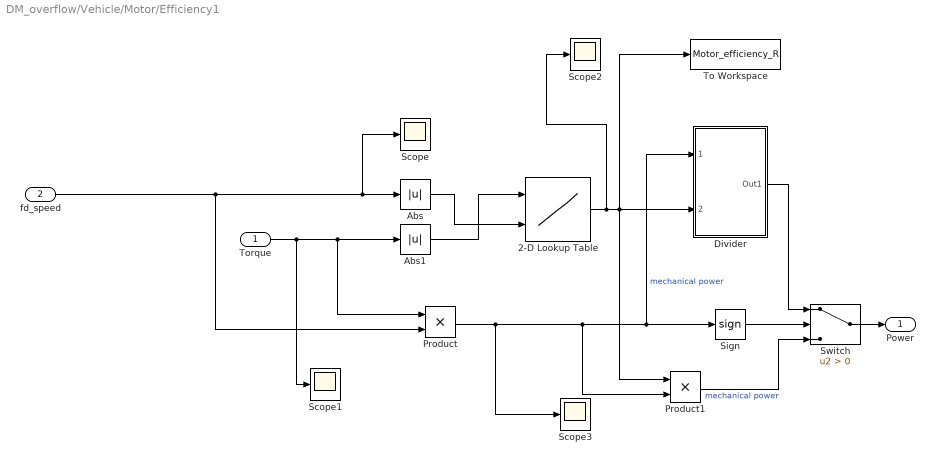
== system DM_overflow/Vehicle/Motor/Efficiency1 ==
  Torque : Inport
  fd_speed : Inport  Port=2
  2-D Lookup Table : Lookup_n-D  BreakpointsForDimension1=efficiency_torque_3D1  BreakpointsForDimension2=efficiency_speed_3D1  Table=efficiency_3D1  InternalRulePriority=Speed  RndMeth=Simplest  InputSameDT=on
      settings: InputPortMap=u0,u1
  Abs : Abs
  Abs1 : Abs
  Divider : Subsystem
  Product : Product
  Product1 : Product
  Scope{,1..3} (4 alike) : Scope
  Sign : Signum
  Switch : Switch  Criteria=u2 > Threshold
  To Workspace : ToWorkspace  VariableName=Motor_efficiency_R  SaveFormat=Timeseries  SampleTime=-1
  Power : Outport
  wires:
  Torque/1 -> Scope1/1, Product/1, Abs1/1
  Product/1 -> Scope3/1, Product1/2, Divider/1(1), Sign/1  "mechanical power"
  Sign/1 -> Switch/2
  Switch/1 -> Power/1
  2-D Lookup Table/1 -> Scope2/1, Product1/1, To Workspace/1, Divider/2(2)
  Product1/1 -> Switch/3  "mechanical power"
  Divider/1(Out1) -> Switch/1
  Abs1/1 -> 2-D Lookup Table/1
  Abs/1 -> 2-D Lookup Table/2
  fd_speed/1 -> Scope/1, Abs/1, Product/2

== system DM_overflow/Vehicle/Motor/Efficiency/Divider ==
  1 : Inport
  2 : Inport  Port=2
  Bus Creator : BusCreator  Inputs=2
  Interpreted MATLAB Function : MATLABFcn  MATLABFcn=myFunction
  Out1 : Outport
  wires:
  1/1 -> Bus Creator/1
  2/1 -> Bus Creator/2
  Bus Creator/1 -> Interpreted MATLAB Function/1
  Interpreted MATLAB Function/1 -> Out1/1

== system DM_overflow/Vehicle/Motor/Efficiency1/Divider ==
  1 : Inport
  2 : Inport  Port=2
  Bus Creator : BusCreator  Inputs=2
  Interpreted MATLAB Function : MATLABFcn  MATLABFcn=myFunction
  Out1 : Outport
  wires:
  1/1 -> Bus Creator/1
  2/1 -> Bus Creator/2
  Bus Creator/1 -> Interpreted MATLAB Function/1
  Interpreted MATLAB Function/1 -> Out1/1
